simulink model "myfilesimu"  (R2022b)
settings: Solver=VariableStepAuto  StartTime=0.0  StopTime=10.0  RelTol=1e-3
settings Model: Creator=wider  LastModifiedBy=wider

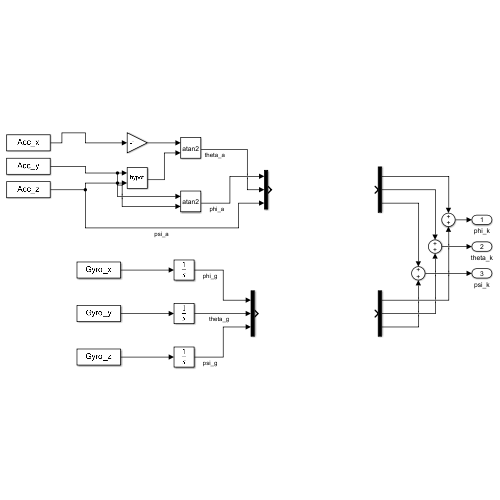
[thumbnail: Simulink's stored preview of the top-level diagram]
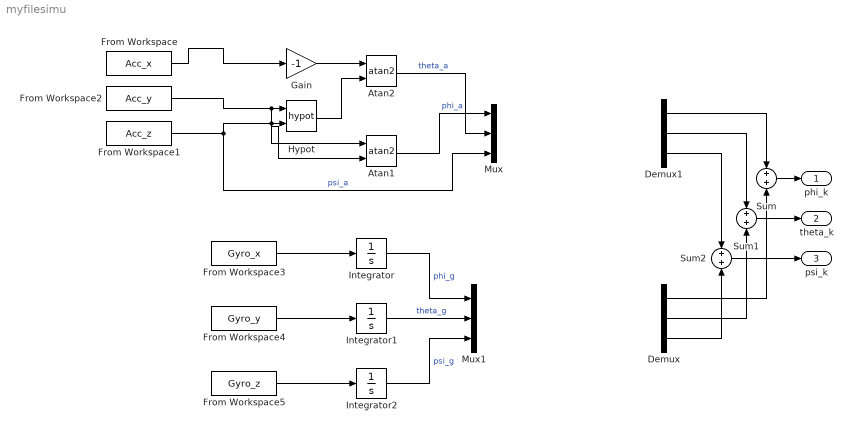
== system myfilesimu ==
  Atan1 : Trigonometry  Operator=atan2
  Atan2 : Trigonometry  Operator=atan2
  Demux : Demux  Outputs=3
  Demux1 : Demux  Outputs=3
  From Workspace : FromWorkspace  VariableName=Acc_x  SampleTime=0.01
  From Workspace1 : FromWorkspace  VariableName=Acc_z  SampleTime=0.01
  From Workspace2 : FromWorkspace  VariableName=Acc_y  SampleTime=0.01
  From Workspace3 : FromWorkspace  VariableName=Gyro_x  SampleTime=0.01
  From Workspace4 : FromWorkspace  VariableName=Gyro_y  SampleTime=0.01
  From Workspace5 : FromWorkspace  VariableName=Gyro_z  SampleTime=0.01
  Gain : Gain  Gain=-1
  Hypot : Math  Operator=hypot
  Integrator : Integrator
  Integrator1 : Integrator
  Integrator2 : Integrator
  Mux : Mux  Inputs=3
  Mux1 : Mux  Inputs=3
  Sum : Sum
  Sum1 : Sum
  Sum2 : Sum
  phi_k : Outport
  theta_k : Outport  Port=2
  psi_k : Outport  Port=3
  wires:
  From Workspace/1 -> Gain/1
  From Workspace2/1 -> Atan1/1, Hypot/1
  From Workspace1/1 -> Mux/3, Atan1/2, Hypot/2  "psi_a"
  Gain/1 -> Atan2/1
  Hypot/1 -> Atan2/2
  Atan1/1 -> Mux/1  "phi_a"
  From Workspace3/1 -> Integrator/1
  From Workspace4/1 -> Integrator1/1
  From Workspace5/1 -> Integrator2/1
  Integrator2/1 -> Mux1/3  "psi_g"
  Integrator1/1 -> Mux1/2  "theta_g"
  Integrator/1 -> Mux1/1  "phi_g"
  Sum/1 -> phi_k/1
  Sum1/1 -> theta_k/1
  Atan2/1 -> Mux/2  "theta_a"
  Demux1/1 -> Sum/1
  Demux/1 -> Sum/2
  Demux1/2 -> Sum1/1
  Demux/2 -> Sum1/2
  Demux/3 -> Sum2/2
  Demux1/3 -> Sum2/1
  Sum2/1 -> psi_k/1
